simulink subsystem "magnetic_sensor"  (R2022b)
settings: Solver=VariableStepAuto  StartTime=0.0  StopTime=10.0  RelTol=1e-3
undefined symbols (not defined in the file or in its folder): sensors
settings Model: Creator=robertopistonenascone  LastModifiedBy=Nicolò

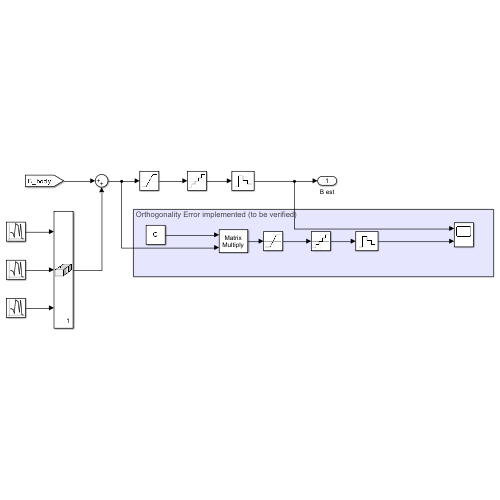
[thumbnail: Simulink's stored preview of the top-level diagram]
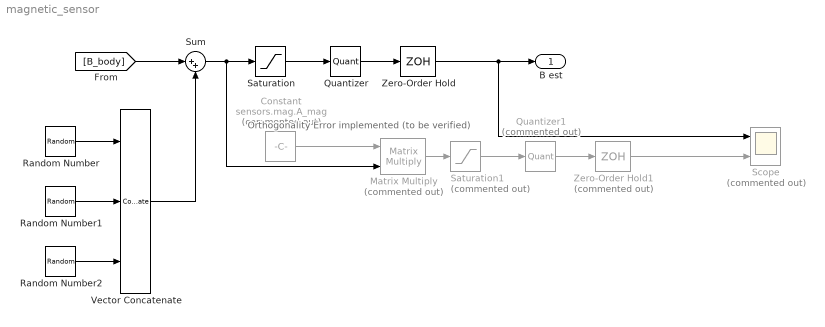
== system magnetic_sensor ==
  note: Orthogonality Error implemented (to be verified)
  Constant : Constant  Commented=on  Value=sensors.mag.A_mag
  Matrix Multiply : Product  Commented=on  Multiplication=Matrix(*)
  Quantizer : Quantizer  QuantizationInterval=sensors.mag.quant_T
  Quantizer1 : Quantizer  Commented=on  QuantizationInterval=sensors.mag.quant_T
  Random Number : RandomNumber  Variance=sensors.mag.variance  SampleTime=0.1
  Random Number1 : RandomNumber  Variance=sensors.mag.variance  Seed=1  SampleTime=0.1
  Random Number2 : RandomNumber  Variance=sensors.mag.variance  Seed=2  SampleTime=0.1
  Saturation : Saturate  UpperLimit=sensors.mag.FMR  LowerLimit=-sensors.mag.FMR
  Saturation1 : Saturate  Commented=on  UpperLimit=sensors.mag.FMR  LowerLimit=-sensors.mag.FMR
  Scope : Scope  Commented=on  NumInputPorts=2
  Sum : Sum  Inputs=|++
  Vector Concatenate : Concatenate  NumInputs=3  Mode=Multidimensional array
  Zero-Order Hold : ZeroOrderHold  SampleTime=sensors.mag.frequency
  Zero-Order Hold1 : ZeroOrderHold  Commented=on  SampleTime=sensors.mag.frequency
  B est : Outport
  wires:
  Sum/1 -> Matrix Multiply/2, Saturation/1
  Random Number/1 -> Vector Concatenate/1
  Random Number1/1 -> Vector Concatenate/2
  Random Number2/1 -> Vector Concatenate/3
  Vector Concatenate/1 -> Sum/2
  Saturation/1 -> Quantizer/1
  Quantizer/1 -> Zero-Order Hold/1
  Zero-Order Hold/1 -> Scope/1, B est/1
  [B_body] -> Sum/1
  Constant/1 -> Matrix Multiply/1
  Zero-Order Hold1/1 -> Scope/2
  Quantizer1/1 -> Zero-Order Hold1/1
  Saturation1/1 -> Quantizer1/1
  Matrix Multiply/1 -> Saturation1/1
